simulink model "Sensor_AirDataPitot"  (R2016b)
settings: Solver=FixedStepAuto  StartTime=0.0  StopTime=10.0  RelTol=1e-3
libraries: Sensors_Lib x4
settings Model: ParameterArgumentNames=sens  Creator=katiekwiz  LastModifiedBy=rega0051

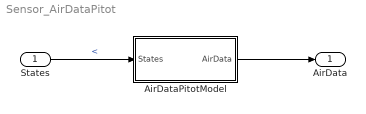
== system Sensor_AirDataPitot ==
  States : Inport  OutDataTypeStr=Bus: States
  AirDataPitotModel : Subsystem  Variant=on
  AirData : Outport  OutDataTypeStr=Bus: AirData
  wires:
  States/1 -> AirDataPitotModel/1(States)  "<"
  AirDataPitotModel/1(AirData) -> AirData/1

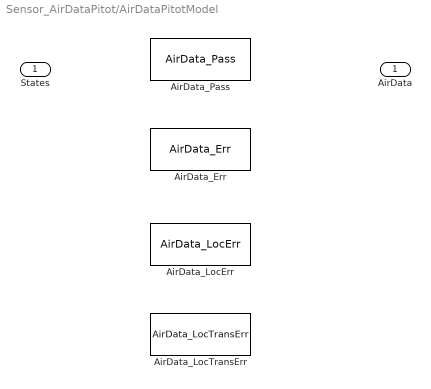
== system Sensor_AirDataPitot/AirDataPitotModel ==
  States : Inport  OutDataTypeStr=Bus: States
  AirData_Err : Sensors_Lib/AirData Sensor Models/AirData_Err  VariantControl=VarAirData_Err
      settings: AttributesFormatString=Variant: %<VariantControl> : %<Variant>
  AirData_LocErr : Sensors_Lib/AirData Sensor Models/AirData_LocErr  VariantControl=VarAirData_LocErr
      settings: AttributesFormatString=Variant: %<VariantControl> : %<Variant>
  AirData_LocTransErr : Sensors_Lib/AirData Sensor Models/AirData_LocTransErr  VariantControl=VarAirData_LocTransErr
      settings: AttributesFormatString=Variant: %<VariantControl> : %<Variant>
  AirData_Pass : Sensors_Lib/AirData Sensor Models/AirData_Pass  VariantControl=VarAirData_Pass
      settings: AttributesFormatString=Variant: %<VariantControl> : %<Variant>
  AirData : Outport  OutDataTypeStr=Bus: AirData
